simulink library "AV_Blocks_Library"  (R2019b)
settings: Solver=VariableStepAuto  StartTime=0.0  StopTime=10.0  RelTol=1e-3
undefined symbols (not defined in the file or in its folder): driving
libraries: drivingscenarioandsensors x3, drivinglib x2
settings Model: Creator=chrst  LastModifiedBy=chrst
settings DataIOCC: ReturnWorkspaceOutputs=off
settings DebuggingCC: ArithmeticOperatorsInVariantConditions=warning
settings SFSimCC: SimUseLocalCustomCode=off  CustomCodeUndefinedFunction=UseInterfaceOnly
settings RTWCC: RTWUseLocalCustomCode=off

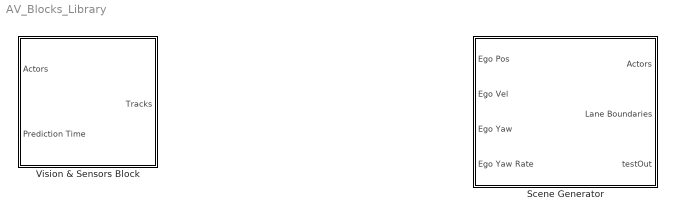
== system AV_Blocks_Library ==
  Scene Generator : Subsystem
  Vision & Sensors Block : Subsystem

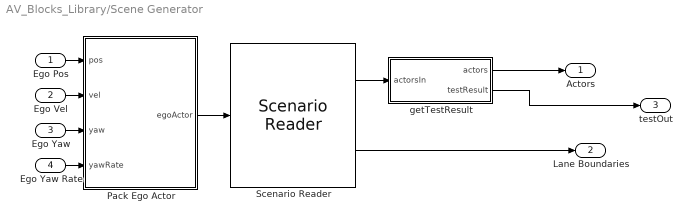
== system AV_Blocks_Library/Scene Generator ==
  Ego Pos : Inport
  Ego Vel : Inport  Port=2
  Ego Yaw : Inport  Port=3
  Ego Yaw Rate : Inport  Port=4
  Pack Ego Actor : MATLAB Function  TreatAsAtomicUnit=on
  Scenario Reader : drivingscenarioandsensors/Scenario Reader  ScenarioSource=From workspace  ScenarioFileName=LFACC_04_Curve_CutInOut.mat  ScenarioVariableName=scenario  OutputCoordinateSystem=Vehicle coordinates  EgoVehicleSource=Input port  EgoVehicleActorID=1  SampleTime=0.1  LaneBoundaryOutput=Ego vehicle lane boundaries  LaneBoundaryDistance=0:0.5:60  LaneBoundaryLocation=Inner edge of lane markings  BusNameSource=Auto  BusName=BusActors  BusName2Source=Auto  BusName2=BusLaneBoundaries  SimulateUsing=Interpreted execution
      settings: SourceProductName=Automated Driving Toolbox
  getTestResult : Subsystem
  Actors : Outport  VectorParamsAs1DForOutWhenUnconnected=off
  Lane Boundaries : Outport  Port=2  VectorParamsAs1DForOutWhenUnconnected=off
  testOut : Outport  Port=3
  wires:
  Scenario Reader/2 -> Lane Boundaries/1
  Pack Ego Actor/1(egoActor) -> Scenario Reader/1
  Ego Yaw Rate/1 -> Pack Ego Actor/4(yawRate)
  Ego Pos/1 -> Pack Ego Actor/1(pos)
  Scenario Reader/1 -> getTestResult/1(actorsIn)
  Ego Vel/1 -> Pack Ego Actor/2(vel)
  Ego Yaw/1 -> Pack Ego Actor/3(yaw)
  getTestResult/1(actors) -> Actors/1
  getTestResult/2(testResult) -> testOut/1

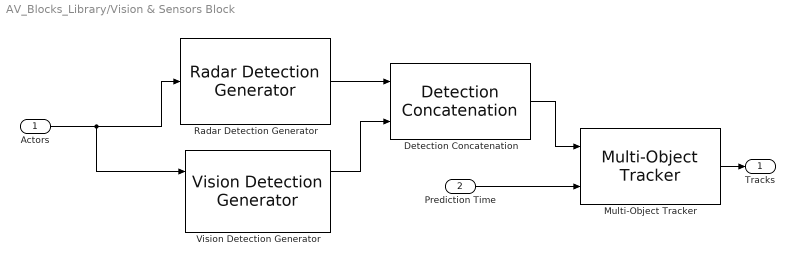
== system AV_Blocks_Library/Vision & Sensors Block ==
  Actors : Inport
  Prediction Time : Inport  Port=2
  Detection Concatenation : drivinglib/Detection Concatenation  NumInputs=2  BusNameSource=Auto  BusName=BusDetectionConcatenation  SimulateUsing=Interpreted execution
      settings: SourceProductName=Automated Driving Toolbox  SourceProductBaseCode=DR
  Multi-Object Tracker : drivinglib/Multi-Object Tracker  FilterInitializationFcn=initcvkf  AssignmentThreshold=30.0  ConfirmationParameters=[ 2, 3 ]  NumCoastingUpdates=5  MaxNumTracks=200  MaxNumSensors=20  TimeInputSource=Input port  HasCostMatrixInput=off  BusNameSource=Auto  BusName=BusMultiObjectTracker  TentativeTracksOutputPort=off  AllTracksOutputPort=off  SimulateUsing=Interpreted execution
      settings: SourceProductName=Automated Driving Toolbox  SourceProductBaseCode=DR
  Radar Detection Generator : drivingscenarioandsensors/Radar Detection Generator  SensorIndex=1  UpdateInterval=0.1  SensorLocation=[ 3.4, 0 ]  Height=0.2  Yaw=0  Pitch=0  Roll=0  BusNameSource=Auto  BusName=BusRadarDetectionGenerator  MaxNumDetectionsSource=Property  MaxNumDetections=50  DetectionCoordinates=Ego Cartesian  SimulateUsing=Interpreted execution  AzimuthResolution=4  ElevationResolution=10  RangeResolution=2.5  RangeRateResolution=0.5  AzimuthBiasFraction=0.1  ElevationBiasFraction=0.1  RangeBiasFraction=0.05  RangeRateBiasFraction=0.05  FieldOfView=[ 20, 5 ]  MaxRange=150  RangeRateLimits=[ -100, 100 ]  DetectionProbability=0.9  FalseAlarmRate=1e-6  ReferenceRange=100  ReferenceRCS=0  HasElevation=off  HasRangeRate=on  HasNoise=on  HasFalseAlarms=on  HasOcclusion=on  InitialSeedSource=Repeatable  InitialSeed=0  UsedSeed=driving.internal.SimulinkUtilities.seedManager(gcb)  ActorProfilesSource=Parameters  ActorProfilesParameters=driving.internal.ActorProfilesRadarParameters  ActorProfilesExpression=struct( 'ClassID', 0, 'Length', 4.7, 'Width', 1.8, 'Height', 1.4, 'OriginOffset', [ -1.35, 0, 0 ], 'RCSPattern', [ 10, 10; 10, 10 ], 'RCSAzimuthAngles', [ -180, 180 ], 'RCSElevationAngles', [ -90, 90 ] )
      settings: SourceProductName=Automated Driving Toolbox  SourceProductBaseCode=DR
  Vision Detection Generator : drivingscenarioandsensors/Vision Detection Generator  SensorIndex=1  DetectorOutput=Lanes and objects  UpdateInterval=0.1  LaneUpdateInterval=0.1  SensorLocation=[ 1.9, 0 ]  Height=1.1  Yaw=0  Pitch=1  Roll=0  BusNameSource=Auto  BusName=BusObjectDetections  BusName2Source=Auto  BusName2=BusLaneDetections  MaxNumDetectionsSource=Property  MaxNumDetections=50  MaxNumLanesSource=Property  MaxNumLanes=30  DetectionCoordinates=Ego Cartesian  SimulateUsing=Interpreted execution  MaxRange=150  BoundingBoxAccuracy=5  ProcessNoiseIntensity=5  MaxSpeed=50  MaxAllowedOcclusion=0.5  MinObjectImageSize=[ 15, 15 ]  DetectionProbability=0.9  FalsePositivesPerImage=0.1  MinLaneImageSize=[ 20, 3 ]  LaneBoundaryAccuracy=3  HasNoise=on  InitialSeedSource=Repeatable  InitialSeed=0  UsedSeed=driving.internal.SimulinkUtilities.seedManager(gcb)  ActorProfilesSource=Parameters  ActorProfilesParameters=driving.internal.ActorProfilesParameters  ActorProfilesExpression=struct( 'ClassID', 0, 'Length', 4.7, 'Width', 1.8, 'Height', 1.4, 'OriginOffset', [ -1.35, 0, 0 ] )  Intrinsics=driving.internal.cameraIntrinsics
      settings: SourceProductName=Automated Driving Toolbox
  Tracks : Outport  VectorParamsAs1DForOutWhenUnconnected=off
  wires:
  Actors/1 -> Vision Detection Generator/1, Radar Detection Generator/1
  Prediction Time/1 -> Multi-Object Tracker/2
  Radar Detection Generator/1 -> Detection Concatenation/1
  Vision Detection Generator/1 -> Detection Concatenation/2
  Detection Concatenation/1 -> Multi-Object Tracker/1
  Multi-Object Tracker/1 -> Tracks/1

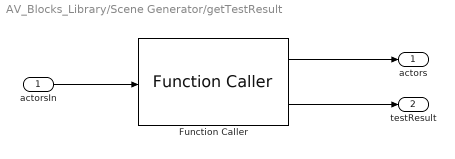
== system AV_Blocks_Library/Scene Generator/getTestResult ==
  actorsIn : Inport
  Function Caller : FunctionCaller  FunctionPrototype=[actors,testOutput] = readActors(actors)  InputArgumentSpecifications=<Enter example>  OutputArgumentSpecifications=<Enter example>
  actors : Outport
  testResult : Outport  Port=2
  wires:
  actorsIn/1 -> Function Caller/1
  Function Caller/1 -> actors/1
  Function Caller/2 -> testResult/1

== matlab function AV_Blocks_Library/Scene Generator/Pack Ego Actor ==
  data: pos input; egoActor output; vel input; yaw input; yawRate input
function egoActor = packEgo(pos,vel,yaw,yawRate)
% Pack ego information into a single ego actor bus
%
% Imoprtant note:
% Output is a bus of type BusActorsActors. This is the same bus used by the
% helperScenarioReader to output an individual actor. If you change the
% output bus name of helperScenarioReader, change the output bus name here
% as well by clicking on 'Edit Data' in the menu above.

egoActor = struct(...
    'ActorID',1,...
    'Position', [pos(1) pos(2) 0], ...
    'Velocity', [vel(1) vel(2) 0], ...
    'Roll', 0, ...
    'Pitch', 0, ...
    'Yaw', yaw, ...
    'AngularVelocity', [0 0 yawRate]);
